simulink model "smartbuilding"  (R2013b)
settings: Solver=ode45  StartTime=0.0  StopTime=10.0  RelTol=1e-3
settings Model: Creator=bboyer  LastModifiedBy=ltraonou
settings DebuggingCC: StateNameClashWarn=warning

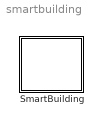
== system smartbuilding ==
  SmartBuilding : Stateflow chart  TreatAsAtomicUnit=on

== stateflow chart smartbuilding/SmartBuilding ==
  state Room
    state Running
    Running -> Running [order 1] : [!need[id] && H[id] == 0 && T[id] <= Tget[id]]
        | {need[id] = true}
    Running -> Running [order 2] : [need[id] & T[id] > Tget[id]]
        | {need[id] = false}
    Running -> Running [order 4] : [cold[id] && T[id] >= Tlow[id]]
        | {cold[id] = false}
    Running -> Running [order 3] : [!cold & T[id] < Tlow[id]]
        | {cold[id]=true}
  state Heater
    state Off
    state On
    Off -> On [order 1] : [T[r] <= Ton[r]]
        | {H[r] = 0} / ON
    Off -> Off [order 2] : MOVE [true]
        | {r = target}
    On -> Off [order 2] : MOVE {h[r] = 0, r = target} / OFF
    On -> Off [order 1] : [T[r] >= Toff[r]]
        | {H[r] = 0} / OFF
  data: id local double =0; r local int32 =0; need constant boolean size=ROOMS; T local double size=ROOMS; Tget constant double size=ROOMS; Tlow local double; T0 constant double size=ROOMS; cold local boolean size=ROOMS; ROOMS constant int32 =3; HEATERS local int32 =2
  events: OFF local FUNCTION_CALL_EVENT; ON local FUNCTION_CALL_EVENT; MOVE local FUNCTION_CALL_EVENT
